simulink model "bai_3"  (R2023a)
settings: Solver=VariableStepAuto  StartTime=0.0  StopTime=10.0  RelTol=1e-3
libraries: dspsrcs4 x4, dspfdesign x3, simulink_extras x1, simulink x1
settings Model: Creator=quoct  LastModifiedBy=Admin

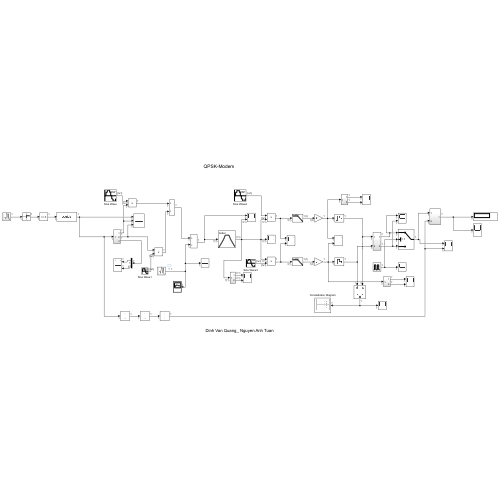
[thumbnail: Simulink's stored preview of the top-level diagram]
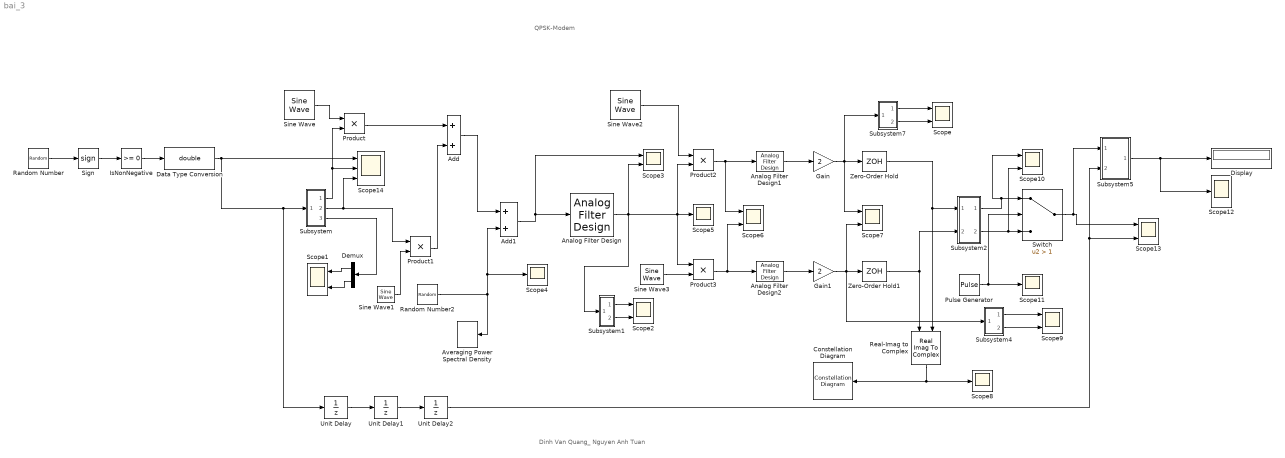
== system bai_3 ==
  note: Dinh Van Quang_ Nguyen Anh Tuan
  note: QPSK-Modem
  Add : Sum
  Add1 : Sum
  Analog Filter Design : dspfdesign/Analog Filter Design  method=Butterworth  filttype=Bandpass  N=8  Wlo=30  Whi=80  Rp=2  Rs=40
  Analog Filter Design1 : dspfdesign/Analog Filter Design  method=Butterworth  filttype=Lowpass  N=8  Wlo=30  Whi=80  Rp=2  Rs=40
  Analog Filter Design2 : dspfdesign/Analog Filter Design  method=Butterworth  filttype=Lowpass  N=8  Wlo=30  Whi=80  Rp=2  Rs=40
  Averaging Power Spectral Density : simulink_extras/Additional Sinks/Averaging Power Spectral Density  npts=128  fftpts=512  HowOften=64  sampleT=0.1
  Constellation Diagram : ConstellationDiagram  WindowPosition=[382.000000,84.000000,600.000000,600.000000,]  ScopeFrameLocation=window
  Data Type Conversion : DataTypeConversion  OutDataTypeStr=double  SaturateOnIntegerOverflow=off  RndMeth=Floor
  Demux : Demux  Outputs=2
  Display : Display
  Gain : Gain  Gain=2
  Gain1 : Gain  Gain=2
  IsNonNegative : simulink/Logic and Bit Operations/Compare To Zero  relop=>=  OutDataTypeStr=boolean
      settings: LibrarySourceBlock=|
      | simulink/Quick Insert/Logic and Bit
      | Operations/IsNonNegative
  Product{,1..3} (4 alike) : Product
  Pulse Generator : DiscretePulseGenerator  PulseType=Time based  Period=10  PulseWidth=5
  Random Number : RandomNumber  SampleTime=0.1
  Random Number2 : RandomNumber  SampleTime=0.1
  Real-Imag to Complex : RealImagToComplex
  Scope{,1..3,6..7,9..10,13} (9 alike) : Scope  NumInputPorts=2
  Scope{4..5,8,11..12} (5 alike) : Scope
  Scope14 : Scope  NumInputPorts=3
  Sign : Signum
  Sine Wave{,1..3} (4 alike) : dspsrcs4/Sine Wave  Amplitude=1  Frequency=100  Phase=0  SampleMode=Discrete  OutComplex=Real  CompMethod=Trigonometric fcn  TableSize=Speed  SampleTime=1/1000  SamplesPerFrame=1  ResetState=Restart at time zero  OutputFrames=off  dataType=double  wordLen=16  udDataType=sfix(16)  fracBitsMode=Best precision  numFracBits=15  OutDataTypeStr=double  LastOutDataTypeStr=double
  Subsystem : Subsystem
  Subsystem1 : Subsystem
  Subsystem2 : Subsystem
  Subsystem4 : Subsystem
  Subsystem5 : Subsystem
  Subsystem7 : Subsystem
  Switch : Switch  Criteria=u2 > Threshold  Threshold=1  SaturateOnIntegerOverflow=off  InputSameDT=off
  Unit Delay : UnitDelay  SampleTime=-1  HasFrameUpgradeWarning=on
  Unit Delay1 : UnitDelay  SampleTime=-1  HasFrameUpgradeWarning=on
  Unit Delay2 : UnitDelay  SampleTime=-1  HasFrameUpgradeWarning=on
  Zero-Order Hold : ZeroOrderHold  SampleTime=-1
  Zero-Order Hold1 : ZeroOrderHold  SampleTime=-1
  wires:
  Unit Delay1/1 -> Unit Delay2/1
  Sine Wave/1 -> Product/1
  Product1/1 -> Add/2
  Product/1 -> Add/1
  Sine Wave1/1 -> Product1/2
  Add/1 -> Add1/1
  Subsystem/3(Out3) -> Demux/1
  Data Type Conversion/1 -> Unit Delay/1, Subsystem/1(In1), Scope14/1
  Analog Filter Design/1 -> Product3/1, Product2/2, Scope5/1, Scope3/2, Subsystem1/1(In1)
  Subsystem1/1(Out1) -> Scope2/1
  Subsystem1/2(Out2) -> Scope2/2
  Product2/1 -> Scope6/1, Analog Filter Design1/1
  Product3/1 -> Scope6/2, Analog Filter Design2/1
  Analog Filter Design2/1 -> Gain1/1
  Analog Filter Design1/1 -> Gain/1
  Gain/1 -> Zero-Order Hold/1, Subsystem7/1(In1), Scope7/1
  Gain1/1 -> Subsystem4/1(In1), Zero-Order Hold1/1, Scope7/2
  Zero-Order Hold1/1 -> Real-Imag to Complex/1, Subsystem2/2(In2)
  Add1/1 -> Scope3/1, Analog Filter Design/1
  Zero-Order Hold/1 -> Real-Imag to Complex/2, Subsystem2/1(In1)
  Pulse Generator/1 -> Scope11/1, Switch/2
  Switch/1 -> Scope13/1, Subsystem5/1(In1)
  Unit Delay2/1 -> Scope13/2, Subsystem5/2(In2)
  Sine Wave2/1 -> Product2/1
  Sine Wave3/1 -> Product3/2
  Unit Delay/1 -> Unit Delay1/1
  IsNonNegative/1 -> Data Type Conversion/1
  Sign/1 -> IsNonNegative/1
  Subsystem/1(Out1) -> Product/2, Scope14/2
  Subsystem/2(Out2) -> Scope14/3, Product1/1
  Random Number2/1 -> Add1/2, Scope4/1, Averaging Power Spectral Density/1
  Random Number/1 -> Sign/1
  Subsystem4/1(Out1) -> Scope9/1
  Subsystem4/2(Out2) -> Scope9/2
  Subsystem2/2(Out2) -> Switch/3, Scope10/2
  Subsystem2/1(Out1) -> Switch/1, Scope10/1
  Subsystem7/1(Out1) -> Scope/1
  Subsystem7/2(Out2) -> Scope/2
  Subsystem5/1(Out1) -> Display/1, Scope12/1
  Demux/1 -> Scope1/1
  Demux/2 -> Scope1/2
  Real-Imag to Complex/1 -> Scope8/1, Constellation Diagram/1

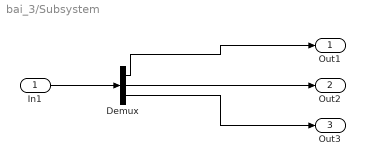
== system bai_3/Subsystem ==
  In1 : Inport
  Demux : Demux  Outputs=3
  Out1 : Outport
  Out2 : Outport  Port=2
  Out3 : Outport  Port=3
  wires:
  In1/1 -> Demux/1
  Demux/1 -> Out1/1
  Demux/2 -> Out2/1
  Demux/3 -> Out3/1

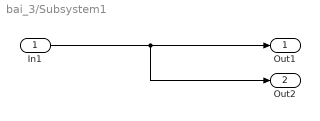
== system bai_3/Subsystem1 ==
  In1 : Inport
  Out1 : Outport
  Out2 : Outport  Port=2
  wires:
  In1/1 -> Out2/1, Out1/1

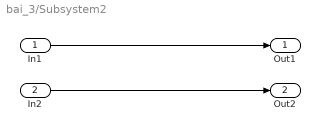
== system bai_3/Subsystem2 ==
  In1 : Inport
  In2 : Inport  Port=2
  Out1 : Outport
  Out2 : Outport  Port=2
  wires:
  In1/1 -> Out1/1
  In2/1 -> Out2/1

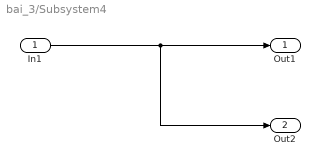
== system bai_3/Subsystem4 ==
  In1 : Inport
  Out1 : Outport
  Out2 : Outport  Port=2
  wires:
  In1/1 -> Out1/1, Out2/1

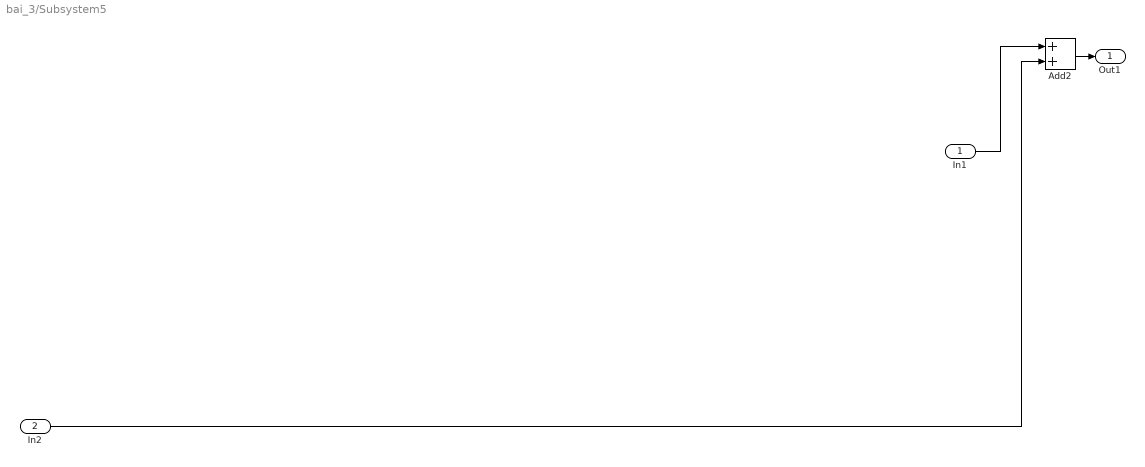
== system bai_3/Subsystem5 ==
  In1 : Inport
  In2 : Inport  Port=2
  Add2 : Sum
  Out1 : Outport
  wires:
  In1/1 -> Add2/1
  In2/1 -> Add2/2
  Add2/1 -> Out1/1

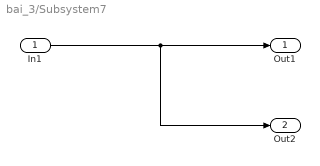
== system bai_3/Subsystem7 ==
  In1 : Inport
  Out1 : Outport
  Out2 : Outport  Port=2
  wires:
  In1/1 -> Out1/1, Out2/1
